simulink model "inverse_GSFR_Individual_Vars"  (R2019b)
settings: Solver=VariableStepAuto  StartTime=0.0  StopTime=20  MaxStep=0.01  RelTol=1e-3
settings Model: Creator=ruiva  LastModifiedBy=ruiva

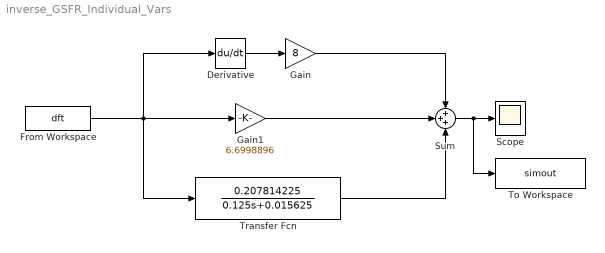
== system inverse_GSFR_Individual_Vars ==
  Derivative : Derivative
  From Workspace : FromWorkspace  VariableName=dft  SampleTime=0
  Gain : Gain  Gain=8
  Gain1 : Gain  Gain=6.6998896
  Scope : Scope
  Sum : Sum  Inputs=+++
  To Workspace : ToWorkspace  VariableName=simout  SaveFormat=Timeseries  SampleTime=-1
  Transfer Fcn : TransferFcn  Numerator=[0.207814225]  Denominator=[0.125 0.015625]
  wires:
  Derivative/1 -> Gain/1
  From Workspace/1 -> Derivative/1, Gain1/1, Transfer Fcn/1
  Transfer Fcn/1 -> Sum/3
  Gain1/1 -> Sum/2
  Gain/1 -> Sum/1
  Sum/1 -> To Workspace/1, Scope/1
